simulink model "atividade4"  (R2024b)
settings: Solver=VariableStepAuto  StartTime=0.0  StopTime=60  RelTol=1e-3
values from neighbouring files (symbols this model uses):
  A = [A1, zeros(3) ... (first row only)    [apc.m]    (also in example1_1.m = [-a_(2:end)', [1; 0]]; script4.m = [1.8 1; -0.8 0])
  B = [B11(2:end), B12(2:end) ... (first row only)    [apc.m]    (also in example1_1.m = b(2:3)'; script4.m = [0.4; 0.6])
  D = [D1, zeros(3,1) ... (first row only)    [apc.m]    (also in example1_1.m = -a_(2:end)'; script4.m = [1.8; -0.8])
  F = zeros(2*N)    [apc.m]    (also in atividade1.m = zeros(N,1); class2.m = zeros(N,1); example1_1.m = zeros(N,length(a)); script4.m = [])
  H = [H1, [0, 0, 0] ... (first row only)    [apc.m]    (also in example1_1.m = [1, 0]; script4.m = [1 0])
  K = K_(1:2,:)    [apc.m]    (also in example1_1.m = K(1,:))
  kr = zeros(2)    [apc.m]    (also in script4.m = sum(k))
  Ts = 0.03    [apc.m]
libraries: cstblocks x2
settings Model: Creator=room2  LastModifiedBy=room2

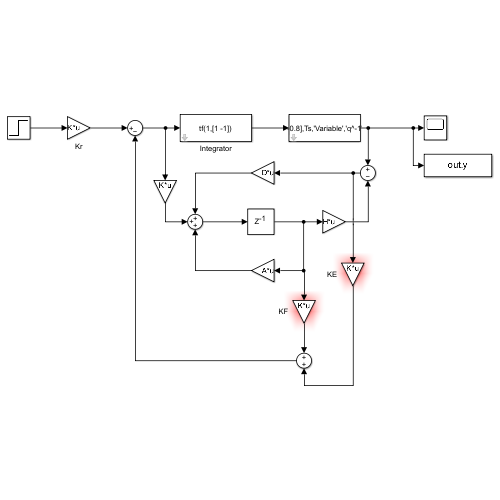
[thumbnail: Simulink's stored preview of the top-level diagram]
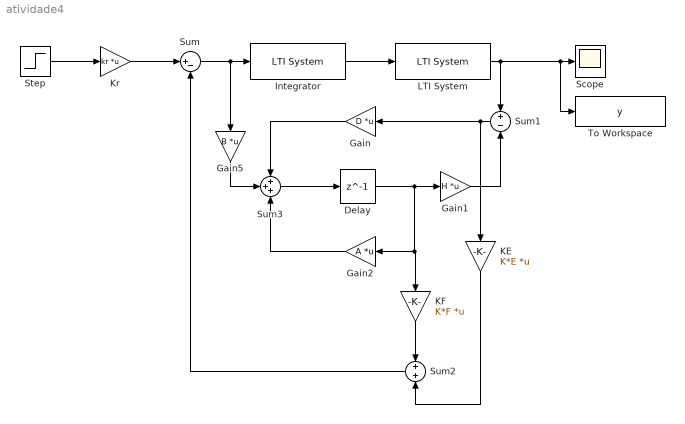
== system atividade4 ==
  Delay : Delay  DelayLength=1
  Gain : Gain  Gain=D  Multiplication=Matrix(K*u)
  Gain1 : Gain  Gain=H  Multiplication=Matrix(K*u)
  Gain2 : Gain  Gain=A  Multiplication=Matrix(K*u)
  Gain5 : Gain  Gain=B  Multiplication=Matrix(K*u)
  Integrator : cstblocks/LTI System  sys=tf(1,[1 -1])  IC=[]  PadeOrder=0
  KE : Gain  Gain=K*E  Multiplication=Matrix(K*u)
  KF : Gain  Gain=K*F  Multiplication=Matrix(K*u)
  Kr : Gain  Gain=kr  Multiplication=Matrix(K*u)
  LTI System : cstblocks/LTI System  sys=tf([0.4 0.6],[1 -0.8],Ts,'Variable','q^-1','IODelay',1);  IC=[]  PadeOrder=0
  Scope : Scope
  Step : Step  Time=0  SampleTime=0
  Sum : Sum  Inputs=|+-
  Sum1 : Sum  Inputs=+|-
  Sum2 : Sum
  Sum3 : Sum  Inputs=+++
  To Workspace : ToWorkspace  VariableName=y  SaveFormat=Timeseries  SampleTime=-1
  wires:
  Step/1 -> Kr/1
  Kr/1 -> Sum/1
  Sum/1 -> Gain5/1, Integrator/1
  Integrator/1 -> LTI System/1
  LTI System/1 -> Sum1/1, To Workspace/1, Scope/1
  Sum1/1 -> Gain/1, KE/1
  Gain1/1 -> Sum1/2
  Delay/1 -> Gain2/1, KF/1, Gain1/1
  KF/1 -> Sum2/1
  KE/1 -> Sum2/2
  Sum3/1 -> Delay/1
  Gain/1 -> Sum3/1
  Gain2/1 -> Sum3/3
  Gain5/1 -> Sum3/2
  Sum2/1 -> Sum/2
